simulink model "FlowChartNotation"  (R2020b)
settings: Solver=VariableStepAuto  StartTime=0.0  StopTime=10.0  RelTol=1e-3
settings Model: Creator=apple  LastModifiedBy=apple

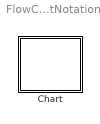
== system FlowChartNotation ==
  Chart : Stateflow chart  TreatAsAtomicUnit=on

== stateflow chart FlowChartNotation/Chart ==
  state A
    en:fprintf("Entry A");
    du:fprintf("During A");
    ex:fprintf("Exit A");
    state A1
      en:fprintf("Entry A1");
      du:fprintf("During A1");
      ex:fprintf("Exit A1");
    state A2
      en:fprintf("Entry A2");
      du:fprintf("During A2");
      ex:fprintf("Exit A2");
    state A3
      en:fprintf("Entry A3");
      du:fprintf("During A3");
      ex:fprintf("Exit A3");
    (junction 10) -> A1 [order 1] : [x> 6]
    (junction 9) -> (junction 9) [order 1] : [x<3]{x = x + 1;}
    (default) -> (junction 3)
    A -> (junction 3) : E_one
    (junction 3) -> (junction 9) : {x = x + 1;}
    (junction 9) -> (junction 10) [order 2]
    (junction 10) -> A2 [order 3]
    (junction 10) -> A3 [order 2] : [x> 4]
  (default) -> A : {x = 0;}
  data: x local
  events: E_one local FUNCTION_CALL_EVENT
